simulink subsystem "susbysmotor"  (R2023b)
settings: Solver=VariableStepAuto  StartTime=0.0  StopTime=10.0  RelTol=1e-3
libraries: arduinolib x6, simulink x2
settings Model: Creator=chaya  LastModifiedBy=Usuario_UMA

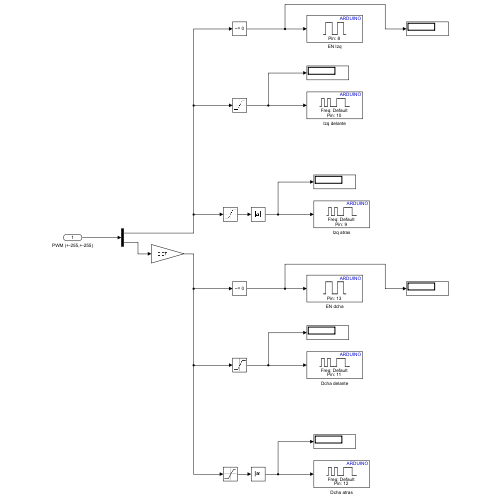
[thumbnail: Simulink's stored preview of the top-level diagram]
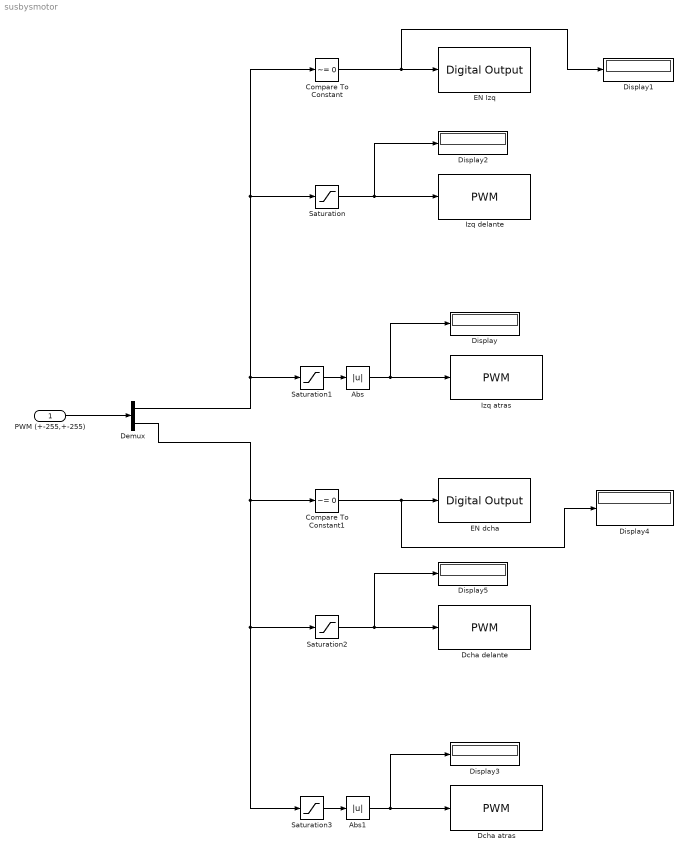
== system susbysmotor ==
  PWM (+-255,+-255) : Inport
  Abs : Abs  SaturateOnIntegerOverflow=off
  Abs1 : Abs  SaturateOnIntegerOverflow=off
  Compare To Constant : simulink/Logic and Bit Operations/Compare To Constant  relop=~=  const=0  OutDataTypeStr=boolean
  Compare To Constant1 : simulink/Logic and Bit Operations/Compare To Constant  relop=~=  const=0  OutDataTypeStr=boolean
  Dcha atras : arduinolib/PWM  pinNumber=12  frequencyType=Default  desiredFrequency=490.2  achievableFrequency=490.2
  Dcha delante : arduinolib/PWM  pinNumber=11  frequencyType=Default  desiredFrequency=490.2  achievableFrequency=490.2
  Demux : Demux  Outputs=2
  Display{,1..5} (6 alike) : Display
  EN Izq : arduinolib/Digital Output  pinNumber=8  Direction=output  blockPlatform=arduino
  EN dcha : arduinolib/Digital Output  pinNumber=13  Direction=output  blockPlatform=arduino
  Izq atras : arduinolib/PWM  pinNumber=10  frequencyType=Default  desiredFrequency=490.2  achievableFrequency=490.2
  Izq delante : arduinolib/PWM  pinNumber=9  frequencyType=Default  desiredFrequency=490.2  achievableFrequency=490.2
  Saturation : Saturate  UpperLimit=255  LowerLimit=0
  Saturation1 : Saturate  UpperLimit=0  LowerLimit=-255
  Saturation2 : Saturate  UpperLimit=255  LowerLimit=0
  Saturation3 : Saturate  UpperLimit=0  LowerLimit=-255
  wires:
  Demux/2 -> Saturation3/1, Saturation2/1, Compare To Constant1/1
  Compare To Constant1/1 -> Display4/1, EN dcha/1
  Saturation3/1 -> Abs1/1
  Saturation2/1 -> Display5/1, Dcha delante/1
  Abs1/1 -> Dcha atras/1, Display3/1
  Saturation1/1 -> Abs/1
  Saturation/1 -> Display2/1, Izq delante/1
  Compare To Constant/1 -> Display1/1, EN Izq/1
  PWM (+-255,+-255)/1 -> Demux/1
  Abs/1 -> Izq atras/1, Display/1
  Demux/1 -> Compare To Constant/1, Saturation/1, Saturation1/1
